simulink model "untitled"  (R2019a)
settings: Solver=VariableStepAuto  StartTime=0.0  StopTime=20  RelTol=1e-3
settings Model: Creator=Qais  LastModifiedBy=Qais

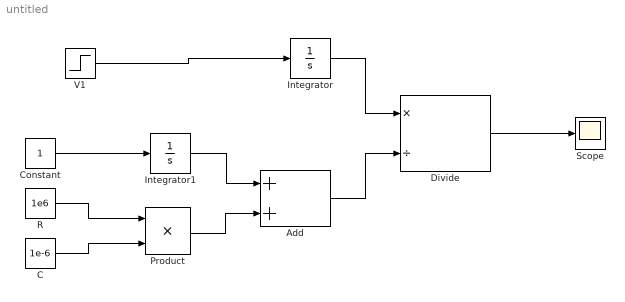
== system untitled ==
  "Add " : Sum
  C : Constant  Value=1e-6
  "Constant " : Constant
  "Divide " : Product  Inputs=*/
  "Integrator " : Integrator
  "Integrator1 " : Integrator
  "Product " : Product
  R : Constant  Value=1e6
  "Scope " : Scope
  V1 : Step  SampleTime=0
  wires:
  "Constant "/1 -> "Integrator1 "/1
  V1/1 -> "Integrator "/1
  R/1 -> "Product "/1
  C/1 -> "Product "/2
  "Integrator1 "/1 -> "Add "/1
  "Product "/1 -> "Add "/2
  "Add "/1 -> "Divide "/2
  "Integrator "/1 -> "Divide "/1
  "Divide "/1 -> "Scope "/1
